simulink subsystem "Magneto1"  (R2021a)
settings: Solver=VariableStepAuto  StartTime=0.0  StopTime=10.0  RelTol=1e-3
undefined symbols (not defined in the file): imu1, Ts
libraries: simulink x4
settings Model: Creator=Laura  LastModifiedBy=Laura

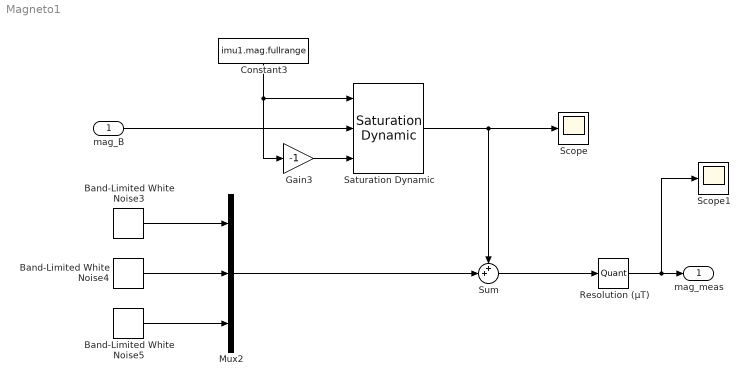
== system Magneto1 ==
  mag_B : Inport
  Band-Limited White Noise3 : simulink/Sources/Band-Limited White Noise  Cov=imu1.mag.noisepower(1)  Ts=Ts  seed=[23341]
  Band-Limited White Noise4 : simulink/Sources/Band-Limited White Noise  Cov=imu1.mag.noisepower(2)  Ts=Ts  seed=[23341]
  Band-Limited White Noise5 : simulink/Sources/Band-Limited White Noise  Cov=imu1.mag.noisepower(3)  Ts=Ts  seed=[23341]
  Constant3 : Constant  Value=imu1.mag.fullrange
  Gain3 : Gain  Gain=-1
  Mux2 : Mux  Inputs=3
  Resolution (μT) : Quantizer  QuantizationInterval=imu1.mag.quantization  LinearizeAsGain=off
  Saturation Dynamic : simulink/Discontinuities/Saturation Dynamic  OutMin=[]  OutMax=[]  OutDataTypeStr=Inherit: Same as second input  OutDataType=fixdt(1, 16)  OutScaling=2^-10  DoSatur=off
  Scope : Scope
  Scope1 : Scope
  Sum : Sum  Inputs=++|
  mag_meas : Outport
  wires:
  Band-Limited White Noise5/1 -> Mux2/3
  Band-Limited White Noise3/1 -> Mux2/1
  Band-Limited White Noise4/1 -> Mux2/2
  Gain3/1 -> Saturation Dynamic/3
  Saturation Dynamic/1 -> Scope/1, Sum/1
  mag_B/1 -> Saturation Dynamic/2
  Constant3/1 -> Gain3/1, Saturation Dynamic/1
  Mux2/1 -> Sum/2
  Sum/1 -> Resolution (μT)/1
  Resolution (μT)/1 -> Scope1/1, mag_meas/1
